simulink model "bai2"  (R2015a)
settings: Solver=ode3  StartTime=0.0  StopTime=10.0  FixedStep=1/1024  RelTol=1e-3
settings Model: Creator=Win 10  LastModifiedBy=Win 10

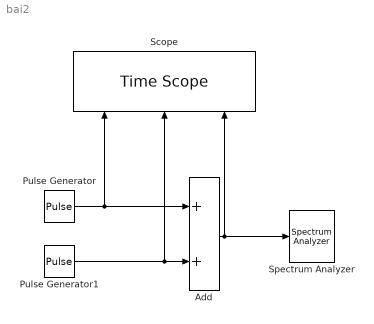
== system bai2 ==
  Add : Sum
  Pulse Generator : DiscretePulseGenerator  Amplitude=2  Period=4096  PulseWidth=1024  SampleTime=1/1024  VectorParams1D=off
  Pulse Generator1 : DiscretePulseGenerator  Period=4096  PulseWidth=1024  PhaseDelay=1024  SampleTime=1/1024
  Scope : TimeScope  NumInputPorts=3
  Spectrum Analyzer : SpectrumAnalyzer
  wires:
  Pulse Generator1/1 -> Scope/2, Add/2
  Pulse Generator/1 -> Scope/1, Add/1
  Add/1 -> Scope/3, Spectrum Analyzer/1
